simulink model "dekf_schaetzung"  (R2021a)
settings: Solver=VariableStepAuto  StartTime=0.0  StopTime=time_est  RelTol=1e-3
values from neighbouring files (symbols this model uses):
  Delta = block.DialogPrm(1).Data    [battery_dual_ekf.m]    (also in last_ekf.m)
settings Model: Creator=saleh  LastModifiedBy=saleh

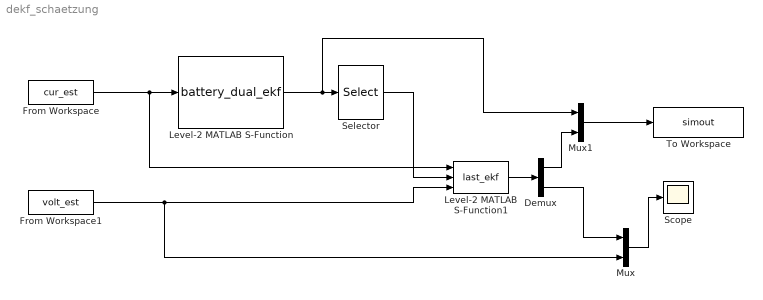
== system dekf_schaetzung ==
  Demux : Demux  Outputs=2
  From Workspace : FromWorkspace  VariableName=cur_est  SampleTime=Delta
  From Workspace1 : FromWorkspace  VariableName=volt_est  SampleTime=Delta
  Level-2 MATLAB S-Function : M-S-Function  FunctionName=battery_dual_ekf  Parameters=Delta, x_0, P_0, x_L_0, P_L_0, a, Z_k, W_k, Z_k, W_L_k, Q_e, Cg
  Level-2 MATLAB S-Function1 : M-S-Function  FunctionName=last_ekf  Parameters=Delta, x_b_0, P_b_0, Z_b_k, W_b_k, Cg
  Mux : Mux  Inputs=2
  Mux1 : Mux  Inputs=2
  Scope : Scope
  Selector : Selector  InputPortWidth=6  IndexOptions=Index vector (dialog)  Indices=[6]  OutputSizes=1
  To Workspace : ToWorkspace  VariableName=simout  SampleTime=-1
  wires:
  From Workspace/1 -> Level-2 MATLAB S-Function1/1, Level-2 MATLAB S-Function/1
  Level-2 MATLAB S-Function/1 -> Mux1/1, Selector/1
  Selector/1 -> Level-2 MATLAB S-Function1/2
  From Workspace1/1 -> Mux/2, Level-2 MATLAB S-Function1/3
  Level-2 MATLAB S-Function1/1 -> Demux/1
  Mux/1 -> Scope/1
  Demux/2 -> Mux/1
  Demux/1 -> Mux1/2
  Mux1/1 -> To Workspace/1
